simulink model "Trot"  (R2025b)
settings: Solver=VariableStepAuto  StartTime=0.0  StopTime=60  RelTol=0.01  AbsTol=0.01  EnableMultiTasking=on
undefined symbols (not defined in the file): a, b, c, X, Y, Z
libraries: sm_lib x58, nesl_utility x37, hdlsllib x12
(part 4 of 4)

== matlab function Trot/RL/MATLAB Function2 ==
  data: t input; q_roll output; leg_id input; q_hip output; q_knee output
function [q_roll, q_hip, q_knee] = motion_walker_v8_extended(t, leg_id)
    % Trot gait — diagonal pairs move together
    %   Group A: RF(0) + LR(2)  phase = 0.0
    %   Group B: LF(1) + RR(3)  phase = 0.5
    
    % ================= Tunables =================
    ang_hip_crouch = deg2rad(30);    % Hip joint crouch angle maintained at 30 degrees
    ang_crouch     = deg2rad(-40);   % Knee joint crouch angle maintained at -40 degrees
    
    % <--- Modification 1: Reduce step size
    hip_swing_amp  = deg2rad(8);
    
    ang_fwd  = ang_hip_crouch - hip_swing_amp;  % 24 degrees
    ang_back = ang_hip_crouch + hip_swing_amp;  % 36 degrees
    
    % <--- Modification 2: Reduce auxiliary motion amplitude to match the smaller step size
    ang_lift       = deg2rad(-5);    % Leg lift bending reduced
    ang_comp       = deg2rad(-6);    % Stance phase compensation reduced
    
    % ================= Timing =================
    T_crouch = 2.0;              
    T_hold   = 3.0;              
    T_ramp   = 2.0;              
    
    % <--- Modification 3: Increase cycle time to make it slower/smoother
    T_cycle  = 1.8;
    duty     = 0.50;             
    
    % ================= Phase offsets =================
    phase_offset = [0.0, 0.5, 0.0, 0.5];
    phi = phase_offset(leg_id + 1);
    
    % ================= Smooth interpolators =================
    smooth = @(x) (1 - cos(x * pi)) / 2;
    bump   = @(x) (1 - cos(2 * x * pi)) / 2;
    
    % ==========================================================
    % Stage 1 & 2: Crouch & Hold
    % ==========================================================
    if t < T_crouch + T_hold
        s = smooth(min(t / T_crouch, 1.0));
        if t >= T_crouch
            s = 1.0;
        end
        q_roll = 0;                          
        q_hip  = s * ang_hip_crouch;
        q_knee = s * ang_crouch;
        return;
    end
    
    % ==========================================================
    % Stage 3: Trot
    % ==========================================================
    t_walk = t - T_crouch - T_hold;
    ramp = smooth(min(t_walk / T_ramp, 1.0));
    phase = mod(t_walk / T_cycle + phi, 1.0);
    
    % --- Full-amplitude trot trajectory ---
    if phase < duty
        % ===== STANCE: foot on ground =====
        % Keep your previously correct direction: ang_back -> ang_fwd
        s = smooth(phase / duty);
        hip_walk  = ang_back + s * (ang_fwd - ang_back); 
        
        % Knee joint compensation (amplitude reduced)
        knee_walk = ang_crouch + sin((phase / duty) * pi) * ang_comp;
        
    else
        % ===== SWING: foot in air =====
        % Keep your previously correct direction: ang_fwd -> ang_back
        s = (phase - duty) / (1.0 - duty);
        hip_walk  = ang_fwd + smooth(s) * (ang_back - ang_fwd);
        knee_walk = ang_crouch + bump(s) * ang_lift;
    end
    
    % --- Blend from rest into trot ---
    q_roll = 0;                              
    q_hip  = ang_hip_crouch + ramp * (hip_walk - ang_hip_crouch);
    q_knee = ang_crouch + ramp * (knee_walk - ang_crouch);
end
